simulink model "test_mdl"  (R2018a)
settings: Solver=VariableStepAuto  StartTime=0.0  StopTime=10.0  RelTol=1e-3
(part 4 of 8)

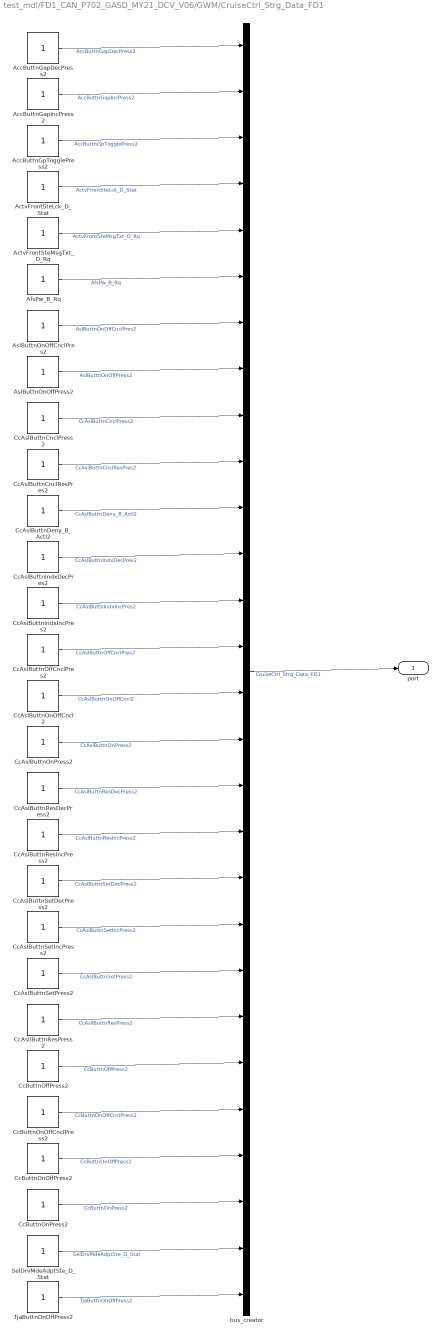
== system test_mdl/FD1_CAN_P702_GASD_MY21_DCV_V06/GWM/CruiseCtrl_Strg_Data_FD1 ==
  AccButtnGapDecPress2 : Constant
  AccButtnGapIncPress2 : Constant
  AccButtnGpTogglePress2 : Constant
  ActvFrontSteLck_D_Stat : Constant
  ActvFrontSteMsgTxt_D_Rq : Constant
  AfsPw_B_Rq : Constant
  AslButtnOnOffCnclPres2 : Constant
  AslButtnOnOffPress2 : Constant
  CcAslButtnCnclPress2 : Constant
  CcAslButtnCnclResPres2 : Constant
  CcAslButtnDeny_B_Actl2 : Constant
  CcAslButtnIndxDecPres2 : Constant
  CcAslButtnIndxIncPres2 : Constant
  CcAslButtnOffCnclPres2 : Constant
  CcAslButtnOnOffCncl2 : Constant
  CcAslButtnOnPress2 : Constant
  CcAslButtnResDecPress2 : Constant
  CcAslButtnResIncPress2 : Constant
  CcAslButtnSetDecPress2 : Constant
  CcAslButtnSetIncPress2 : Constant
  CcAslButtnSetPress2 : Constant
  CcAsllButtnResPress2 : Constant
  CcButtnOffPress2 : Constant
  CcButtnOnOffCnclPress2 : Constant
  CcButtnOnOffPress2 : Constant
  CcButtnOnPress2 : Constant
  SelDrvMdeAdptSte_D_Stat : Constant
  TjaButtnOnOffPress2 : Constant
  bus_creator : BusCreator  Inputs=28
  port : Outport
  wires:
  bus_creator/1 -> port/1  "CruiseCtrl_Strg_Data_FD1"
  AccButtnGapDecPress2/1 -> bus_creator/1  "AccButtnGapDecPress2"
  AccButtnGapIncPress2/1 -> bus_creator/2  "AccButtnGapIncPress2"
  AccButtnGpTogglePress2/1 -> bus_creator/3  "AccButtnGpTogglePress2"
  ActvFrontSteLck_D_Stat/1 -> bus_creator/4  "ActvFrontSteLck_D_Stat"
  ActvFrontSteMsgTxt_D_Rq/1 -> bus_creator/5  "ActvFrontSteMsgTxt_D_Rq"
  AfsPw_B_Rq/1 -> bus_creator/6  "AfsPw_B_Rq"
  AslButtnOnOffCnclPres2/1 -> bus_creator/7  "AslButtnOnOffCnclPres2"
  AslButtnOnOffPress2/1 -> bus_creator/8  "AslButtnOnOffPress2"
  CcAslButtnCnclPress2/1 -> bus_creator/9  "CcAslButtnCnclPress2"
  CcAslButtnCnclResPres2/1 -> bus_creator/10  "CcAslButtnCnclResPres2"
  CcAslButtnDeny_B_Actl2/1 -> bus_creator/11  "CcAslButtnDeny_B_Actl2"
  CcAslButtnIndxDecPres2/1 -> bus_creator/12  "CcAslButtnIndxDecPres2"
  CcAslButtnIndxIncPres2/1 -> bus_creator/13  "CcAslButtnIndxIncPres2"
  CcAslButtnOffCnclPres2/1 -> bus_creator/14  "CcAslButtnOffCnclPres2"
  CcAslButtnOnOffCncl2/1 -> bus_creator/15  "CcAslButtnOnOffCncl2"
  CcAslButtnOnPress2/1 -> bus_creator/16  "CcAslButtnOnPress2"
  CcAslButtnResDecPress2/1 -> bus_creator/17  "CcAslButtnResDecPress2"
  CcAslButtnResIncPress2/1 -> bus_creator/18  "CcAslButtnResIncPress2"
  CcAslButtnSetDecPress2/1 -> bus_creator/19  "CcAslButtnSetDecPress2"
  CcAslButtnSetIncPress2/1 -> bus_creator/20  "CcAslButtnSetIncPress2"
  CcAslButtnSetPress2/1 -> bus_creator/21  "CcAslButtnSetPress2"
  CcAsllButtnResPress2/1 -> bus_creator/22  "CcAsllButtnResPress2"
  CcButtnOffPress2/1 -> bus_creator/23  "CcButtnOffPress2"
  CcButtnOnOffCnclPress2/1 -> bus_creator/24  "CcButtnOnOffCnclPress2"
  CcButtnOnOffPress2/1 -> bus_creator/25  "CcButtnOnOffPress2"
  CcButtnOnPress2/1 -> bus_creator/26  "CcButtnOnPress2"
  SelDrvMdeAdptSte_D_Stat/1 -> bus_creator/27  "SelDrvMdeAdptSte_D_Stat"
  TjaButtnOnOffPress2/1 -> bus_creator/28  "TjaButtnOnOffPress2"

== system test_mdl/FD1_CAN_P702_GASD_MY21_DCV_V06/GWM/DCACA_Data1_FD1 ==
  CoolFanDcac_D_Rq : Constant
  DcacAcUDetct_B_Falt : Constant
  DcacBp1BrkrOpn_B_Falt : Constant
  DcacBp2BrkrOpn_B_Falt : Constant
  DcacClntFlw_D_Rq : Constant
  DcacErr_B_Stat : Constant
  DcacGfci_B_Falt : Constant
  DcacIpRcBrkrOpn_B_Falt : Constant
  DcacOverTe_B_Falt : Constant
  DcacOvrld_B_Falt : Constant
  DcacPlugPrsnt_B_Stat : Constant
  DcacRdy_D2_Stat : Constant
  DcacRdy_D_Stat : Constant
  bus_creator : BusCreator  Inputs=13
  port : Outport
  wires:
  bus_creator/1 -> port/1  "DCACA_Data1_FD1"
  CoolFanDcac_D_Rq/1 -> bus_creator/1  "CoolFanDcac_D_Rq"
  DcacAcUDetct_B_Falt/1 -> bus_creator/2  "DcacAcUDetct_B_Falt"
  DcacBp1BrkrOpn_B_Falt/1 -> bus_creator/3  "DcacBp1BrkrOpn_B_Falt"
  DcacBp2BrkrOpn_B_Falt/1 -> bus_creator/4  "DcacBp2BrkrOpn_B_Falt"
  DcacClntFlw_D_Rq/1 -> bus_creator/5  "DcacClntFlw_D_Rq"
  DcacErr_B_Stat/1 -> bus_creator/6  "DcacErr_B_Stat"
  DcacGfci_B_Falt/1 -> bus_creator/7  "DcacGfci_B_Falt"
  DcacIpRcBrkrOpn_B_Falt/1 -> bus_creator/8  "DcacIpRcBrkrOpn_B_Falt"
  DcacOverTe_B_Falt/1 -> bus_creator/9  "DcacOverTe_B_Falt"
  DcacOvrld_B_Falt/1 -> bus_creator/10  "DcacOvrld_B_Falt"
  DcacPlugPrsnt_B_Stat/1 -> bus_creator/11  "DcacPlugPrsnt_B_Stat"
  DcacRdy_D2_Stat/1 -> bus_creator/12  "DcacRdy_D2_Stat"
  DcacRdy_D_Stat/1 -> bus_creator/13  "DcacRdy_D_Stat"

== system test_mdl/FD1_CAN_P702_GASD_MY21_DCV_V06/GWM/DCACA_Data2_FD1 ==
  DcacIn_I_Actl : Constant
  DcacIn_U2_Actl : Constant
  DcacIn_U_Actl : Constant
  Dcac_Te_Actl : Constant
  bus_creator : BusCreator  Inputs=4
  port : Outport
  wires:
  bus_creator/1 -> port/1  "DCACA_Data2_FD1"
  DcacIn_I_Actl/1 -> bus_creator/1  "DcacIn_I_Actl"
  DcacIn_U2_Actl/1 -> bus_creator/2  "DcacIn_U2_Actl"
  DcacIn_U_Actl/1 -> bus_creator/3  "DcacIn_U_Actl"
  Dcac_Te_Actl/1 -> bus_creator/4  "Dcac_Te_Actl"

== system test_mdl/FD1_CAN_P702_GASD_MY21_DCV_V06/GWM/DCACA_Data3_FD1 ==
  DcacIn_Pw_Mx : Constant
  DcacOut1_Pw_Actl : Constant
  DcacOut2_Pw_Actl : Constant
  DcacOut_Pw_Mx : Constant
  bus_creator : BusCreator  Inputs=4
  port : Outport
  wires:
  bus_creator/1 -> port/1  "DCACA_Data3_FD1"
  DcacIn_Pw_Mx/1 -> bus_creator/1  "DcacIn_Pw_Mx"
  DcacOut1_Pw_Actl/1 -> bus_creator/2  "DcacOut1_Pw_Actl"
  DcacOut2_Pw_Actl/1 -> bus_creator/3  "DcacOut2_Pw_Actl"
  DcacOut_Pw_Mx/1 -> bus_creator/4  "DcacOut_Pw_Mx"

== system test_mdl/FD1_CAN_P702_GASD_MY21_DCV_V06/GWM/DTE_ECGtoHPCM ==
  DteCldBattULo_Eff_Actl : Constant
  DteCldClimt_Eff_Actl : Constant
  DteCldDcac_B_Stat : Constant
  DteCldDrv_Eff_Actl : Constant
  DteCldExtTe_B_Stat : Constant
  DteCldExt_Eff_Actl : Constant
  DteCldId_No_Actl : Constant
  DteCldPayload_B_Stat : Constant
  DteCldRoute_B_Stat : Constant
  DteCldTerrain_B_Stat : Constant
  DteCldTraffic_B_Stat : Constant
  DteCldTrip_L_Actl : Constant
  DteCldTrlrOff_B_Stat : Constant
  DteCldTrlrOn_B_Stat : Constant
  bus_creator : BusCreator  Inputs=14
  port : Outport
  wires:
  bus_creator/1 -> port/1  "DTE_ECGtoHPCM"
  DteCldBattULo_Eff_Actl/1 -> bus_creator/1  "DteCldBattULo_Eff_Actl"
  DteCldClimt_Eff_Actl/1 -> bus_creator/2  "DteCldClimt_Eff_Actl"
  DteCldDcac_B_Stat/1 -> bus_creator/3  "DteCldDcac_B_Stat"
  DteCldDrv_Eff_Actl/1 -> bus_creator/4  "DteCldDrv_Eff_Actl"
  DteCldExtTe_B_Stat/1 -> bus_creator/5  "DteCldExtTe_B_Stat"
  DteCldExt_Eff_Actl/1 -> bus_creator/6  "DteCldExt_Eff_Actl"
  DteCldId_No_Actl/1 -> bus_creator/7  "DteCldId_No_Actl"
  DteCldPayload_B_Stat/1 -> bus_creator/8  "DteCldPayload_B_Stat"
  DteCldRoute_B_Stat/1 -> bus_creator/9  "DteCldRoute_B_Stat"
  DteCldTerrain_B_Stat/1 -> bus_creator/10  "DteCldTerrain_B_Stat"
  DteCldTraffic_B_Stat/1 -> bus_creator/11  "DteCldTraffic_B_Stat"
  DteCldTrip_L_Actl/1 -> bus_creator/12  "DteCldTrip_L_Actl"
  DteCldTrlrOff_B_Stat/1 -> bus_creator/13  "DteCldTrlrOff_B_Stat"
  DteCldTrlrOn_B_Stat/1 -> bus_creator/14  "DteCldTrlrOn_B_Stat"

== system test_mdl/FD1_CAN_P702_GASD_MY21_DCV_V06/GWM/Driver_Dr_Stat_FD1 ==
  BLISLEDStatDriverSide : Constant
  ChildLckFdbckRd_B_Stat : Constant
  ChildLckPw_D_Rq : Constant
  ChildLckPw_N_Cnt : Constant
  Driver_Lock_Sw_Cnt : Constant
  Driver_Lock_Sw_Stat : Constant
  KeyCylSwDrvDr_D_Stat : Constant
  RollCodeDrvDrKeyCyl : Constant
  RvrseMirrorChime_B_Rq : Constant
  WndwDrvSide_D_Stat : Constant
  bus_creator : BusCreator  Inputs=10
  port : Outport
  wires:
  bus_creator/1 -> port/1  "Driver_Dr_Stat_FD1"
  BLISLEDStatDriverSide/1 -> bus_creator/1  "BLISLEDStatDriverSide"
  ChildLckFdbckRd_B_Stat/1 -> bus_creator/2  "ChildLckFdbckRd_B_Stat"
  ChildLckPw_D_Rq/1 -> bus_creator/3  "ChildLckPw_D_Rq"
  ChildLckPw_N_Cnt/1 -> bus_creator/4  "ChildLckPw_N_Cnt"
  Driver_Lock_Sw_Cnt/1 -> bus_creator/5  "Driver_Lock_Sw_Cnt"
  Driver_Lock_Sw_Stat/1 -> bus_creator/6  "Driver_Lock_Sw_Stat"
  KeyCylSwDrvDr_D_Stat/1 -> bus_creator/7  "KeyCylSwDrvDr_D_Stat"
  RollCodeDrvDrKeyCyl/1 -> bus_creator/8  "RollCodeDrvDrKeyCyl"
  RvrseMirrorChime_B_Rq/1 -> bus_creator/9  "RvrseMirrorChime_B_Rq"
  WndwDrvSide_D_Stat/1 -> bus_creator/10  "WndwDrvSide_D_Stat"

== system test_mdl/FD1_CAN_P702_GASD_MY21_DCV_V06/GWM/Dsp_Request_Signals11_FD1 ==
  ApaMdeStat_D_RqDrv : Constant
  ApaSwtch_D_RqMnu : Constant
  CamAutoTowbarZoom : Constant
  CamraOvrlDyn_D_Rq : Constant
  CamraOvrlStat_D_Rq : Constant
  CamraViewSplit_B_Rq : Constant
  CamraZoomMan_D_Rq : Constant
  DistanceBarSetting : Constant
  PrkAidSwtch_D_RqMnu : Constant
  bus_creator : BusCreator  Inputs=9
  port : Outport
  wires:
  bus_creator/1 -> port/1  "Dsp_Request_Signals11_FD1"
  ApaMdeStat_D_RqDrv/1 -> bus_creator/1  "ApaMdeStat_D_RqDrv"
  ApaSwtch_D_RqMnu/1 -> bus_creator/2  "ApaSwtch_D_RqMnu"
  CamAutoTowbarZoom/1 -> bus_creator/3  "CamAutoTowbarZoom"
  CamraOvrlDyn_D_Rq/1 -> bus_creator/4  "CamraOvrlDyn_D_Rq"
  CamraOvrlStat_D_Rq/1 -> bus_creator/5  "CamraOvrlStat_D_Rq"
  CamraViewSplit_B_Rq/1 -> bus_creator/6  "CamraViewSplit_B_Rq"
  CamraZoomMan_D_Rq/1 -> bus_creator/7  "CamraZoomMan_D_Rq"
  DistanceBarSetting/1 -> bus_creator/8  "DistanceBarSetting"
  PrkAidSwtch_D_RqMnu/1 -> bus_creator/9  "PrkAidSwtch_D_RqMnu"

== system test_mdl/FD1_CAN_P702_GASD_MY21_DCV_V06/GWM/ECG_Data2_FD1 ==
  DataMntrSustn_B_Rq : Constant
  DgtlCommPncReset_B_Req : Constant
  PwSustnRdata_B_RqTelem : Constant
  bus_creator : BusCreator  Inputs=3
  port : Outport
  wires:
  bus_creator/1 -> port/1  "ECG_Data2_FD1"
  DataMntrSustn_B_Rq/1 -> bus_creator/1  "DataMntrSustn_B_Rq"
  DgtlCommPncReset_B_Req/1 -> bus_creator/2  "DgtlCommPncReset_B_Req"
  PwSustnRdata_B_RqTelem/1 -> bus_creator/3  "PwSustnRdata_B_RqTelem"

== system test_mdl/FD1_CAN_P702_GASD_MY21_DCV_V06/GWM/ECG_Data3_FD1 ==
  BattULoChrg_D_RqOta : Constant
  CanMsg375_No_Cnt : Constant
  CanMsg375_No_Crc : Constant
  OtaActv_D_Stat : Constant
  VehOnRqstr_D_Stat : Constant
  VehOn_D_RqCld : Constant
  VehStrtInhbt_D_Dsply : Constant
  VehStrtInhbt_D_RqCld : Constant
  VehStrtInhbt_T_Dsply : Constant
  bus_creator : BusCreator  Inputs=9
  port : Outport
  wires:
  bus_creator/1 -> port/1  "ECG_Data3_FD1"
  BattULoChrg_D_RqOta/1 -> bus_creator/1  "BattULoChrg_D_RqOta"
  CanMsg375_No_Cnt/1 -> bus_creator/2  "CanMsg375_No_Cnt"
  CanMsg375_No_Crc/1 -> bus_creator/3  "CanMsg375_No_Crc"
  OtaActv_D_Stat/1 -> bus_creator/4  "OtaActv_D_Stat"
  VehOnRqstr_D_Stat/1 -> bus_creator/5  "VehOnRqstr_D_Stat"
  VehOn_D_RqCld/1 -> bus_creator/6  "VehOn_D_RqCld"
  VehStrtInhbt_D_Dsply/1 -> bus_creator/7  "VehStrtInhbt_D_Dsply"
  VehStrtInhbt_D_RqCld/1 -> bus_creator/8  "VehStrtInhbt_D_RqCld"
  VehStrtInhbt_T_Dsply/1 -> bus_creator/9  "VehStrtInhbt_T_Dsply"

== system test_mdl/FD1_CAN_P702_GASD_MY21_DCV_V06/GWM/ECG_Data4_FD1 ==
  PtWakeupActv1_B_Rq : Constant
  bus_creator : BusCreator  Inputs=1
  port : Outport
  wires:
  bus_creator/1 -> port/1  "ECG_Data4_FD1"
  PtWakeupActv1_B_Rq/1 -> bus_creator/1  "PtWakeupActv1_B_Rq"

== system test_mdl/FD1_CAN_P702_GASD_MY21_DCV_V06/GWM/ECG_Data_FD1 ==
  ChrgrPncEnbl_D_Rq : Constant
  ChrgrPncSustn_B_Rq : Constant
  ExtLghtDsply_B_StatArb : Constant
  ExtLghtFront_D_RqOta : Constant
  ExtLghtLeft_D_RqOta : Constant
  ExtLghtRear_D_RqOta : Constant
  ExtLghtRight_D_RqOta : Constant
  NtfyDrvSocLvl1_Pc_Rq : Constant
  NtfyDrvTrgtDist_L_Rq : Constant
  OBCCSerial_D_Rq : Constant
  PtRmtRprt_D_Stat : Constant
  TlghtTest_D_RqArb : Constant
  bus_creator : BusCreator  Inputs=12
  port : Outport
  wires:
  bus_creator/1 -> port/1  "ECG_Data_FD1"
  ChrgrPncEnbl_D_Rq/1 -> bus_creator/1  "ChrgrPncEnbl_D_Rq"
  ChrgrPncSustn_B_Rq/1 -> bus_creator/2  "ChrgrPncSustn_B_Rq"
  ExtLghtDsply_B_StatArb/1 -> bus_creator/3  "ExtLghtDsply_B_StatArb"
  ExtLghtFront_D_RqOta/1 -> bus_creator/4  "ExtLghtFront_D_RqOta"
  ExtLghtLeft_D_RqOta/1 -> bus_creator/5  "ExtLghtLeft_D_RqOta"
  ExtLghtRear_D_RqOta/1 -> bus_creator/6  "ExtLghtRear_D_RqOta"
  ExtLghtRight_D_RqOta/1 -> bus_creator/7  "ExtLghtRight_D_RqOta"
  NtfyDrvSocLvl1_Pc_Rq/1 -> bus_creator/8  "NtfyDrvSocLvl1_Pc_Rq"
  NtfyDrvTrgtDist_L_Rq/1 -> bus_creator/9  "NtfyDrvTrgtDist_L_Rq"
  OBCCSerial_D_Rq/1 -> bus_creator/10  "OBCCSerial_D_Rq"
  PtRmtRprt_D_Stat/1 -> bus_creator/11  "PtRmtRprt_D_Stat"
  TlghtTest_D_RqArb/1 -> bus_creator/12  "TlghtTest_D_RqArb"

== system test_mdl/FD1_CAN_P702_GASD_MY21_DCV_V06/GWM/ElecHorizon_Data1_FD1 ==
  EhData1_No_Actl : Constant
  bus_creator : BusCreator  Inputs=1
  port : Outport
  wires:
  bus_creator/1 -> port/1  "ElecHorizon_Data1_FD1"
  EhData1_No_Actl/1 -> bus_creator/1  "EhData1_No_Actl"

== system test_mdl/FD1_CAN_P702_GASD_MY21_DCV_V06/GWM/ElecHorizon_Data2_FD1 ==
  EhData2_No_Actl : Constant
  bus_creator : BusCreator  Inputs=1
  port : Outport
  wires:
  bus_creator/1 -> port/1  "ElecHorizon_Data2_FD1"
  EhData2_No_Actl/1 -> bus_creator/1  "EhData2_No_Actl"

== system test_mdl/FD1_CAN_P702_GASD_MY21_DCV_V06/GWM/FourByFourSwitchData_FD1 ==
  AwdMde_D_RqDrv : Constant
  DrvSlipCtlMde_B_Rq3 : Constant
  HdcSwtchPos_B_Actl : Constant
  HybMdeSwtch_B_Rq : Constant
  RearDiffLck_D_RqDrv : Constant
  TrailCtlSwtch_B_Stat3 : Constant
  bus_creator : BusCreator  Inputs=6
  port : Outport
  wires:
  bus_creator/1 -> port/1  "FourByFourSwitchData_FD1"
  AwdMde_D_RqDrv/1 -> bus_creator/1  "AwdMde_D_RqDrv"
  DrvSlipCtlMde_B_Rq3/1 -> bus_creator/2  "DrvSlipCtlMde_B_Rq3"
  HdcSwtchPos_B_Actl/1 -> bus_creator/3  "HdcSwtchPos_B_Actl"
  HybMdeSwtch_B_Rq/1 -> bus_creator/4  "HybMdeSwtch_B_Rq"
  RearDiffLck_D_RqDrv/1 -> bus_creator/5  "RearDiffLck_D_RqDrv"
  TrailCtlSwtch_B_Stat3/1 -> bus_creator/6  "TrailCtlSwtch_B_Stat3"

== system test_mdl/FD1_CAN_P702_GASD_MY21_DCV_V06/GWM/GGCC_Config_Mgmt_ID_1_FD1 ==
  VehicleGGCCData : Constant
  bus_creator : BusCreator  Inputs=1
  port : Outport
  wires:
  bus_creator/1 -> port/1  "GGCC_Config_Mgmt_ID_1_FD1"
  VehicleGGCCData/1 -> bus_creator/1  "VehicleGGCCData"

== system test_mdl/FD1_CAN_P702_GASD_MY21_DCV_V06/GWM/GWM_AutoSar_NetMgmt_FD1 ==
  GWM_AutoSarNMControl : Constant
  GWM_AutoSarNMNodeId : Constant
  GWM_AutoSarNMReserved{1..4} (4 alike) : Constant
  GWM_GWNMProxy : Constant
  GWM_GWOnBoardTester : Constant
  bus_creator : BusCreator  Inputs=8
  port : Outport
  wires:
  bus_creator/1 -> port/1  "GWM_AutoSar_NetMgmt_FD1"
  GWM_AutoSarNMControl/1 -> bus_creator/1  "GWM_AutoSarNMControl"
  GWM_AutoSarNMNodeId/1 -> bus_creator/2  "GWM_AutoSarNMNodeId"
  GWM_AutoSarNMReserved1/1 -> bus_creator/3  "GWM_AutoSarNMReserved1"
  GWM_AutoSarNMReserved2/1 -> bus_creator/4  "GWM_AutoSarNMReserved2"
  GWM_AutoSarNMReserved3/1 -> bus_creator/5  "GWM_AutoSarNMReserved3"
  GWM_AutoSarNMReserved4/1 -> bus_creator/6  "GWM_AutoSarNMReserved4"
  GWM_GWNMProxy/1 -> bus_creator/7  "GWM_GWNMProxy"
  GWM_GWOnBoardTester/1 -> bus_creator/8  "GWM_GWOnBoardTester"

== system test_mdl/FD1_CAN_P702_GASD_MY21_DCV_V06/GWM/Gear_Shift_by_Wire_2_FD1 ==
  GearButtnStuck_B_Actl : Constant
  GsmSrvcRqd_B_Rq : Constant
  TrnGearPwmFalt_B_Actl : Constant
  bus_creator : BusCreator  Inputs=3
  port : Outport
  wires:
  bus_creator/1 -> port/1  "Gear_Shift_by_Wire_2_FD1"
  GearButtnStuck_B_Actl/1 -> bus_creator/1  "GearButtnStuck_B_Actl"
  GsmSrvcRqd_B_Rq/1 -> bus_creator/2  "GsmSrvcRqd_B_Rq"
  TrnGearPwmFalt_B_Actl/1 -> bus_creator/3  "TrnGearPwmFalt_B_Actl"

== system test_mdl/FD1_CAN_P702_GASD_MY21_DCV_V06/GWM/Gear_Shift_by_Wire_FD1 ==
  BrkSwtchPos_B_ActlGsm : Constant
  DrQltyDrv_D_StatGsm : Constant
  GsmGearMsgTxt_D_Rq : Constant
  PrkBrkActv_D_RqGsmGear : Constant
  TrnBtsiOvrrd_B_Stat : Constant
  TrnGearButtn_B_ActlD0 : Constant
  TrnGearButtn_B_ActlD1 : Constant
  TrnGearButtn_B_ActlD2 : Constant
  TrnGearButtn_B_ActlM0 : Constant
  TrnGearButtn_B_ActlM1 : Constant
  TrnGearButtn_B_ActlM2 : Constant
  TrnGearButtn_B_ActlN0 : Constant
  TrnGearButtn_B_ActlN1 : Constant
  TrnGearButtn_B_ActlN2 : Constant
  TrnGearButtn_B_ActlP0 : Constant
  TrnGearButtn_B_ActlP1 : Constant
  TrnGearButtn_B_ActlP2 : Constant
  TrnGearButtn_B_ActlR0 : Constant
  TrnGearButtn_B_ActlR1 : Constant
  TrnGearButtn_B_ActlR2 : Constant
  TrnGearButtn_U_Actl : Constant
  TrnGearRqCnt_B_Actl : Constant
  TrnGear_D_RqDrv : Constant
  TrnGear_No_Cnt : Constant
  TrnGear_No_Cs : Constant
  TrnGsmNtmState_D_Actl : Constant
  TrnRng_D_RqGsm : Constant
  TrnValidGearRq_D_Stat : Constant
  bus_creator : BusCreator  Inputs=28
  port : Outport
  wires:
  bus_creator/1 -> port/1  "Gear_Shift_by_Wire_FD1"
  BrkSwtchPos_B_ActlGsm/1 -> bus_creator/1  "BrkSwtchPos_B_ActlGsm"
  DrQltyDrv_D_StatGsm/1 -> bus_creator/2  "DrQltyDrv_D_StatGsm"
  GsmGearMsgTxt_D_Rq/1 -> bus_creator/3  "GsmGearMsgTxt_D_Rq"
  PrkBrkActv_D_RqGsmGear/1 -> bus_creator/4  "PrkBrkActv_D_RqGsmGear"
  TrnBtsiOvrrd_B_Stat/1 -> bus_creator/5  "TrnBtsiOvrrd_B_Stat"
  TrnGearButtn_B_ActlD0/1 -> bus_creator/6  "TrnGearButtn_B_ActlD0"
  TrnGearButtn_B_ActlD1/1 -> bus_creator/7  "TrnGearButtn_B_ActlD1"
  TrnGearButtn_B_ActlD2/1 -> bus_creator/8  "TrnGearButtn_B_ActlD2"
  TrnGearButtn_B_ActlM0/1 -> bus_creator/9  "TrnGearButtn_B_ActlM0"
  TrnGearButtn_B_ActlM1/1 -> bus_creator/10  "TrnGearButtn_B_ActlM1"
  TrnGearButtn_B_ActlM2/1 -> bus_creator/11  "TrnGearButtn_B_ActlM2"
  TrnGearButtn_B_ActlN0/1 -> bus_creator/12  "TrnGearButtn_B_ActlN0"
  TrnGearButtn_B_ActlN1/1 -> bus_creator/13  "TrnGearButtn_B_ActlN1"
  TrnGearButtn_B_ActlN2/1 -> bus_creator/14  "TrnGearButtn_B_ActlN2"
  TrnGearButtn_B_ActlP0/1 -> bus_creator/15  "TrnGearButtn_B_ActlP0"
  TrnGearButtn_B_ActlP1/1 -> bus_creator/16  "TrnGearButtn_B_ActlP1"
  TrnGearButtn_B_ActlP2/1 -> bus_creator/17  "TrnGearButtn_B_ActlP2"
  TrnGearButtn_B_ActlR0/1 -> bus_creator/18  "TrnGearButtn_B_ActlR0"
  TrnGearButtn_B_ActlR1/1 -> bus_creator/19  "TrnGearButtn_B_ActlR1"
  TrnGearButtn_B_ActlR2/1 -> bus_creator/20  "TrnGearButtn_B_ActlR2"
  TrnGearButtn_U_Actl/1 -> bus_creator/21  "TrnGearButtn_U_Actl"
  TrnGearRqCnt_B_Actl/1 -> bus_creator/22  "TrnGearRqCnt_B_Actl"
  TrnGear_D_RqDrv/1 -> bus_creator/23  "TrnGear_D_RqDrv"
  TrnGear_No_Cnt/1 -> bus_creator/24  "TrnGear_No_Cnt"
  TrnGear_No_Cs/1 -> bus_creator/25  "TrnGear_No_Cs"
  TrnGsmNtmState_D_Actl/1 -> bus_creator/26  "TrnGsmNtmState_D_Actl"
  TrnRng_D_RqGsm/1 -> bus_creator/27  "TrnRng_D_RqGsm"
  TrnValidGearRq_D_Stat/1 -> bus_creator/28  "TrnValidGearRq_D_Stat"

== system test_mdl/FD1_CAN_P702_GASD_MY21_DCV_V06/GWM/GlobalClock_Data_FD1 ==
  GlblClkDay_No_Actl : Constant
  GlblClkHr_No_Actl : Constant
  GlblClkMnte_No_Actl : Constant
  GlblClkScnd_No_Actl : Constant
  GlblClkYr_No_Actl : Constant
  bus_creator : BusCreator  Inputs=5
  port : Outport
  wires:
  bus_creator/1 -> port/1  "GlobalClock_Data_FD1"
  GlblClkDay_No_Actl/1 -> bus_creator/1  "GlblClkDay_No_Actl"
  GlblClkHr_No_Actl/1 -> bus_creator/2  "GlblClkHr_No_Actl"
  GlblClkMnte_No_Actl/1 -> bus_creator/3  "GlblClkMnte_No_Actl"
  GlblClkScnd_No_Actl/1 -> bus_creator/4  "GlblClkScnd_No_Actl"
  GlblClkYr_No_Actl/1 -> bus_creator/5  "GlblClkYr_No_Actl"

== system test_mdl/FD1_CAN_P702_GASD_MY21_DCV_V06/GWM/Global_PATS_Cntrl_Info_FD1 ==
  bus_creator : BusCreator  Inputs=2
  immoControlCmd_T1 : Constant
  immoControlData_T1 : Constant
  port : Outport
  wires:
  bus_creator/1 -> port/1  "Global_PATS_Cntrl_Info_FD1"
  immoControlCmd_T1/1 -> bus_creator/1  "immoControlCmd_T1"
  immoControlData_T1/1 -> bus_creator/2  "immoControlData_T1"

== system test_mdl/FD1_CAN_P702_GASD_MY21_DCV_V06/GWM/Global_PATS_Ctrl_Info2_FD1 ==
  bus_creator : BusCreator  Inputs=2
  immoControlCmd_T2 : Constant
  immoControlData_T2 : Constant
  port : Outport
  wires:
  bus_creator/1 -> port/1  "Global_PATS_Ctrl_Info2_FD1"
  immoControlCmd_T2/1 -> bus_creator/1  "immoControlCmd_T2"
  immoControlData_T2/1 -> bus_creator/2  "immoControlData_T2"

== system test_mdl/FD1_CAN_P702_GASD_MY21_DCV_V06/GWM/HeadUpDisplayReq_FD1 ==
  SelDrvMdeCnfm_D_Stat : Constant
  bus_creator : BusCreator  Inputs=1
  port : Outport
  wires:
  bus_creator/1 -> port/1  "HeadUpDisplayReq_FD1"
  SelDrvMdeCnfm_D_Stat/1 -> bus_creator/1  "SelDrvMdeCnfm_D_Stat"

== system test_mdl/FD1_CAN_P702_GASD_MY21_DCV_V06/GWM/IPC_Infotainment_FD1 ==
  BeltminderAudioMute : Constant
  Chime_Source : Constant
  HdcOn_B_Rq : Constant
  IPC_Attn_Info_Audio : Constant
  IPC_MyKeyVolLimit_St : Constant
  IPC_New_Attn_Event : Constant
  Power_Up_Chime_Modules : Constant
  Veh_V2_Dsply : Constant
  bus_creator : BusCreator  Inputs=8
  port : Outport
  wires:
  bus_creator/1 -> port/1  "IPC_Infotainment_FD1"
  BeltminderAudioMute/1 -> bus_creator/1  "BeltminderAudioMute"
  Chime_Source/1 -> bus_creator/2  "Chime_Source"
  HdcOn_B_Rq/1 -> bus_creator/3  "HdcOn_B_Rq"
  IPC_Attn_Info_Audio/1 -> bus_creator/4  "IPC_Attn_Info_Audio"
  IPC_MyKeyVolLimit_St/1 -> bus_creator/5  "IPC_MyKeyVolLimit_St"
  IPC_New_Attn_Event/1 -> bus_creator/6  "IPC_New_Attn_Event"
  Power_Up_Chime_Modules/1 -> bus_creator/7  "Power_Up_Chime_Modules"
  Veh_V2_Dsply/1 -> bus_creator/8  "Veh_V2_Dsply"

== system test_mdl/FD1_CAN_P702_GASD_MY21_DCV_V06/GWM/IPC_Send_Signals_2_FD1 ==
  ElLongTerm_L_Dsply : Constant
  ElTrip_L_Dsply : Constant
  FuelRange_L_Dsply : Constant
  bus_creator : BusCreator  Inputs=3
  port : Outport
  wires:
  bus_creator/1 -> port/1  "IPC_Send_Signals_2_FD1"
  ElLongTerm_L_Dsply/1 -> bus_creator/1  "ElLongTerm_L_Dsply"
  ElTrip_L_Dsply/1 -> bus_creator/2  "ElTrip_L_Dsply"
  FuelRange_L_Dsply/1 -> bus_creator/3  "FuelRange_L_Dsply"

== system test_mdl/FD1_CAN_P702_GASD_MY21_DCV_V06/GWM/LocationServices_3_FD1 ==
  LocationServices_3 : Constant
  bus_creator : BusCreator  Inputs=1
  port : Outport
  wires:
  bus_creator/1 -> port/1  "LocationServices_3_FD1"
  LocationServices_3/1 -> bus_creator/1  "LocationServices_3"

== system test_mdl/FD1_CAN_P702_GASD_MY21_DCV_V06/GWM/LocationServices_Data1_FD1 ==
  LocationServices_1 : Constant
  bus_creator : BusCreator  Inputs=1
  port : Outport
  wires:
  bus_creator/1 -> port/1  "LocationServices_Data1_FD1"
  LocationServices_1/1 -> bus_creator/1  "LocationServices_1"

== system test_mdl/FD1_CAN_P702_GASD_MY21_DCV_V06/GWM/Locking_Systems_2_FD1 ==
  ChildLckMde_B_Stat : Constant
  ChildLck_D_Dsply : Constant
  DrTgateExtSwMde_B_Stat : Constant
  DrTgateOpen_B_Rq : Constant
  FobComm_D_Stat : Constant
  Keyfob_Pad_Msg_Count : Constant
  L_Pwr_Sliding_Dr_Rqst : Constant
  LockInhibit : Constant
  Lockmsgtxt_D_Rq : Constant
  Power_Decklid_Rqst : Constant
  Power_Liftgate_Rqst : Constant
  R_Pwr_Sliding_Dr_Rqst : Constant
  Remote_Device_Feedback : Constant
  RollCodeUnlock : Constant
  VehLckInd_D_Rq : Constant
  Veh_Lock_EvNum : Constant
  Veh_Lock_Requestor : Constant
  Veh_Lock_Status : Constant
  Veh_Lock_Sub_Id : Constant
  WindowLockout_B_Stat : Constant
  bus_creator : BusCreator  Inputs=20
  port : Outport
  wires:
  bus_creator/1 -> port/1  "Locking_Systems_2_FD1"
  ChildLckMde_B_Stat/1 -> bus_creator/1  "ChildLckMde_B_Stat"
  ChildLck_D_Dsply/1 -> bus_creator/2  "ChildLck_D_Dsply"
  DrTgateExtSwMde_B_Stat/1 -> bus_creator/3  "DrTgateExtSwMde_B_Stat"
  DrTgateOpen_B_Rq/1 -> bus_creator/4  "DrTgateOpen_B_Rq"
  FobComm_D_Stat/1 -> bus_creator/5  "FobComm_D_Stat"
  Keyfob_Pad_Msg_Count/1 -> bus_creator/6  "Keyfob_Pad_Msg_Count"
  L_Pwr_Sliding_Dr_Rqst/1 -> bus_creator/7  "L_Pwr_Sliding_Dr_Rqst"
  LockInhibit/1 -> bus_creator/8  "LockInhibit"
  Lockmsgtxt_D_Rq/1 -> bus_creator/9  "Lockmsgtxt_D_Rq"
  Power_Decklid_Rqst/1 -> bus_creator/10  "Power_Decklid_Rqst"
  Power_Liftgate_Rqst/1 -> bus_creator/11  "Power_Liftgate_Rqst"
  R_Pwr_Sliding_Dr_Rqst/1 -> bus_creator/12  "R_Pwr_Sliding_Dr_Rqst"
  Remote_Device_Feedback/1 -> bus_creator/13  "Remote_Device_Feedback"
  RollCodeUnlock/1 -> bus_creator/14  "RollCodeUnlock"
  VehLckInd_D_Rq/1 -> bus_creator/15  "VehLckInd_D_Rq"
  Veh_Lock_EvNum/1 -> bus_creator/16  "Veh_Lock_EvNum"
  Veh_Lock_Requestor/1 -> bus_creator/17  "Veh_Lock_Requestor"
  Veh_Lock_Status/1 -> bus_creator/18  "Veh_Lock_Status"
  Veh_Lock_Sub_Id/1 -> bus_creator/19  "Veh_Lock_Sub_Id"
  WindowLockout_B_Stat/1 -> bus_creator/20  "WindowLockout_B_Stat"

== system test_mdl/FD1_CAN_P702_GASD_MY21_DCV_V06/GWM/MasterReset_HS3_ECGDat_FD1 ==
  DrvBhavWarn_B_Rq : Constant
  FactoryReset_St : Constant
  KeyOffPwMde_D_Stat : Constant
  ModemReset_D_Stat : Constant
  OfbChrgSetSync_D_Rq : Constant
  bus_creator : BusCreator  Inputs=5
  port : Outport
  wires:
  bus_creator/1 -> port/1  "MasterReset_HS3_ECGDat_FD1"
  DrvBhavWarn_B_Rq/1 -> bus_creator/1  "DrvBhavWarn_B_Rq"
  FactoryReset_St/1 -> bus_creator/2  "FactoryReset_St"
  KeyOffPwMde_D_Stat/1 -> bus_creator/3  "KeyOffPwMde_D_Stat"
  ModemReset_D_Stat/1 -> bus_creator/4  "ModemReset_D_Stat"
  OfbChrgSetSync_D_Rq/1 -> bus_creator/5  "OfbChrgSetSync_D_Rq"

== system test_mdl/FD1_CAN_P702_GASD_MY21_DCV_V06/GWM/Mc_Send_Signals_2_FD1 ==
  AwdRnge_D_ActlIpc : Constant
  BalrMde_D_Rq : Constant
  BalrSwtch_D_Stat : Constant
  BttOn_B_Rq : Constant
  Btt_L_Actl : Constant
  DrvInputRequired_B_Rq : Constant
  EdmSailMde_B_RqDrv : Constant
  EngExhMdeQuiet_D2_Rq : Constant
  EsaOn_B_Rq : Constant
  Mc_VehLangUsrSel_St : Constant
  Mc_VehTimeFrmtUsrSel_St : Constant
  Mc_VehUnitTempUsrSel_St : Constant
  Mc_VehUntTrpCoUsrSel_St : Constant
  Running_Board_Cmd : Constant
  SelDrvMdeDsply_B_Avail : Constant
  SelDrvMdeTxtReset_B_Rq : Constant
  WaitToStartLamp_D_Falt : Constant
  bus_creator : BusCreator  Inputs=17
  port : Outport
  wires:
  bus_creator/1 -> port/1  "Mc_Send_Signals_2_FD1"
  AwdRnge_D_ActlIpc/1 -> bus_creator/1  "AwdRnge_D_ActlIpc"
  BalrMde_D_Rq/1 -> bus_creator/2  "BalrMde_D_Rq"
  BalrSwtch_D_Stat/1 -> bus_creator/3  "BalrSwtch_D_Stat"
  BttOn_B_Rq/1 -> bus_creator/4  "BttOn_B_Rq"
  Btt_L_Actl/1 -> bus_creator/5  "Btt_L_Actl"
  DrvInputRequired_B_Rq/1 -> bus_creator/6  "DrvInputRequired_B_Rq"
  EdmSailMde_B_RqDrv/1 -> bus_creator/7  "EdmSailMde_B_RqDrv"
  EngExhMdeQuiet_D2_Rq/1 -> bus_creator/8  "EngExhMdeQuiet_D2_Rq"
  EsaOn_B_Rq/1 -> bus_creator/9  "EsaOn_B_Rq"
  Mc_VehLangUsrSel_St/1 -> bus_creator/10  "Mc_VehLangUsrSel_St"
  Mc_VehTimeFrmtUsrSel_St/1 -> bus_creator/11  "Mc_VehTimeFrmtUsrSel_St"
  Mc_VehUnitTempUsrSel_St/1 -> bus_creator/12  "Mc_VehUnitTempUsrSel_St"
  Mc_VehUntTrpCoUsrSel_St/1 -> bus_creator/13  "Mc_VehUntTrpCoUsrSel_St"
  Running_Board_Cmd/1 -> bus_creator/14  "Running_Board_Cmd"
  SelDrvMdeDsply_B_Avail/1 -> bus_creator/15  "SelDrvMdeDsply_B_Avail"
  SelDrvMdeTxtReset_B_Rq/1 -> bus_creator/16  "SelDrvMdeTxtReset_B_Rq"
  WaitToStartLamp_D_Falt/1 -> bus_creator/17  "WaitToStartLamp_D_Falt"

== system test_mdl/FD1_CAN_P702_GASD_MY21_DCV_V06/GWM/OTAFuncGWM_ECG_FD1 ==
  OTAFuncGWM_ECG : Constant
  bus_creator : BusCreator  Inputs=1
  port : Outport
  wires:
  bus_creator/1 -> port/1  "OTAFuncGWM_ECG_FD1"
  OTAFuncGWM_ECG/1 -> bus_creator/1  "OTAFuncGWM_ECG"

== system test_mdl/FD1_CAN_P702_GASD_MY21_DCV_V06/GWM/OTAPhysGWM_ECGtoABS ==
  OTAPhysGWM_ECGtoABS : Constant
  bus_creator : BusCreator  Inputs=1
  port : Outport
  wires:
  bus_creator/1 -> port/1  "OTAPhysGWM_ECGtoABS"
  OTAPhysGWM_ECGtoABS/1 -> bus_creator/1  "OTAPhysGWM_ECGtoABS"

== system test_mdl/FD1_CAN_P702_GASD_MY21_DCV_V06/GWM/OTAPhysGWM_ECGtoCCM ==
  OTAPhysGWM_ECGtoCCM : Constant
  bus_creator : BusCreator  Inputs=1
  port : Outport
  wires:
  bus_creator/1 -> port/1  "OTAPhysGWM_ECGtoCCM"
  OTAPhysGWM_ECGtoCCM/1 -> bus_creator/1  "OTAPhysGWM_ECGtoCCM"

== system test_mdl/FD1_CAN_P702_GASD_MY21_DCV_V06/GWM/OTAPhysGWM_ECGtoIPMA ==
  OTAPhysGWM_ECGtoIPMA : Constant
  bus_creator : BusCreator  Inputs=1
  port : Outport
  wires:
  bus_creator/1 -> port/1  "OTAPhysGWM_ECGtoIPMA"
  OTAPhysGWM_ECGtoIPMA/1 -> bus_creator/1  "OTAPhysGWM_ECGtoIPMA"

== system test_mdl/FD1_CAN_P702_GASD_MY21_DCV_V06/GWM/OTAPhysGWM_ECGtoPCM ==
  OTAPhysGWM_ECGtoPCM : Constant
  bus_creator : BusCreator  Inputs=1
  port : Outport
  wires:
  bus_creator/1 -> port/1  "OTAPhysGWM_ECGtoPCM"
  OTAPhysGWM_ECGtoPCM/1 -> bus_creator/1  "OTAPhysGWM_ECGtoPCM"

== system test_mdl/FD1_CAN_P702_GASD_MY21_DCV_V06/GWM/OTAPhysGWM_ECGtoSOBDMC_FD1 ==
  OTAPhysGWM_ECGtoHPCM : Constant
  bus_creator : BusCreator  Inputs=1
  port : Outport
  wires:
  bus_creator/1 -> port/1  "OTAPhysGWM_ECGtoSOBDMC_FD1"
  OTAPhysGWM_ECGtoHPCM/1 -> bus_creator/1  "OTAPhysGWM_ECGtoHPCM"

== system test_mdl/FD1_CAN_P702_GASD_MY21_DCV_V06/GWM/OTAPhysGWM_ECGtoSODCMC ==
  OTAPhysGWM_ECGtoSODCMC : Constant
  bus_creator : BusCreator  Inputs=1
  port : Outport
  wires:
  bus_creator/1 -> port/1  "OTAPhysGWM_ECGtoSODCMC"
  OTAPhysGWM_ECGtoSODCMC/1 -> bus_creator/1  "OTAPhysGWM_ECGtoSODCMC"

== system test_mdl/FD1_CAN_P702_GASD_MY21_DCV_V06/GWM/OTAPhysGWM_ECGtoSODCMD ==
  OTAPhysGWM_ECGtoSODCMD : Constant
  bus_creator : BusCreator  Inputs=1
  port : Outport
  wires:
  bus_creator/1 -> port/1  "OTAPhysGWM_ECGtoSODCMD"
  OTAPhysGWM_ECGtoSODCMD/1 -> bus_creator/1  "OTAPhysGWM_ECGtoSODCMD"

== system test_mdl/FD1_CAN_P702_GASD_MY21_DCV_V06/GWM/OTAPhysGWM_ECGtoSODL ==
  OTAPhysGWM_ECGtoSODL : Constant
  bus_creator : BusCreator  Inputs=1
  port : Outport
  wires:
  bus_creator/1 -> port/1  "OTAPhysGWM_ECGtoSODL"
  OTAPhysGWM_ECGtoSODL/1 -> bus_creator/1  "OTAPhysGWM_ECGtoSODL"

== system test_mdl/FD1_CAN_P702_GASD_MY21_DCV_V06/GWM/OTAPhysGWM_ECGtoSODR ==
  OTAPhysGWM_ECGtoSODR : Constant
  bus_creator : BusCreator  Inputs=1
  port : Outport
  wires:
  bus_creator/1 -> port/1  "OTAPhysGWM_ECGtoSODR"
  OTAPhysGWM_ECGtoSODR/1 -> bus_creator/1  "OTAPhysGWM_ECGtoSODR"

== system test_mdl/FD1_CAN_P702_GASD_MY21_DCV_V06/GWM/OffBrdChrg_Signals ==
  OfbChrgLocIdTrgt_No_Rq : Constant
  OfbChrgLocIdUns_B_Rq : Constant
  OfbChrgPrflWkdy_No_Rq : Constant
  OfbChrgPrflWknd_No_Rq : Constant
  OfbChrgSetDelete_B_Rq : Constant
  OfbChrgSetNow_D_Rq : Constant
  OfbChrgToPcWkdy_D_Actl : Constant
  OfbChrgToPcWknd_D_Actl : Constant
  bus_creator : BusCreator  Inputs=8
  port : Outport
  wires:
  bus_creator/1 -> port/1  "OffBrdChrg_Signals"
  OfbChrgLocIdTrgt_No_Rq/1 -> bus_creator/1  "OfbChrgLocIdTrgt_No_Rq"
  OfbChrgLocIdUns_B_Rq/1 -> bus_creator/2  "OfbChrgLocIdUns_B_Rq"
  OfbChrgPrflWkdy_No_Rq/1 -> bus_creator/3  "OfbChrgPrflWkdy_No_Rq"
  OfbChrgPrflWknd_No_Rq/1 -> bus_creator/4  "OfbChrgPrflWknd_No_Rq"
  OfbChrgSetDelete_B_Rq/1 -> bus_creator/5  "OfbChrgSetDelete_B_Rq"
  OfbChrgSetNow_D_Rq/1 -> bus_creator/6  "OfbChrgSetNow_D_Rq"
  OfbChrgToPcWkdy_D_Actl/1 -> bus_creator/7  "OfbChrgToPcWkdy_D_Actl"
  OfbChrgToPcWknd_D_Actl/1 -> bus_creator/8  "OfbChrgToPcWknd_D_Actl"

== system test_mdl/FD1_CAN_P702_GASD_MY21_DCV_V06/GWM/OffBrdChrg_Signals2 ==
  OfbChrgClearAll_B_Rq : Constant
  OfbChrgGoTDelete_B_Rq : Constant
  OfbChrgGoTElement_D_Rq : Constant
  OfbChrgGoTExtHtr_D_Rq : Constant
  OfbChrgGoTHr_T_Rq : Constant
  OfbChrgGoTMnte_D_Rq : Constant
  OfbChrgGoTOn_D_Rq : Constant
  OfbChrgGoTPrcond_D_Rq : Constant
  OfbChrgGoTTouch_D_Rq : Constant
  OfbChrgGoTUpdate_B_Rq : Constant
  OfbChrgPrflUpdate_B_Rq : Constant
  bus_creator : BusCreator  Inputs=11
  port : Outport
  wires:
  bus_creator/1 -> port/1  "OffBrdChrg_Signals2"
  OfbChrgClearAll_B_Rq/1 -> bus_creator/1  "OfbChrgClearAll_B_Rq"
  OfbChrgGoTDelete_B_Rq/1 -> bus_creator/2  "OfbChrgGoTDelete_B_Rq"
  OfbChrgGoTElement_D_Rq/1 -> bus_creator/3  "OfbChrgGoTElement_D_Rq"
  OfbChrgGoTExtHtr_D_Rq/1 -> bus_creator/4  "OfbChrgGoTExtHtr_D_Rq"
  OfbChrgGoTHr_T_Rq/1 -> bus_creator/5  "OfbChrgGoTHr_T_Rq"
  OfbChrgGoTMnte_D_Rq/1 -> bus_creator/6  "OfbChrgGoTMnte_D_Rq"
  OfbChrgGoTOn_D_Rq/1 -> bus_creator/7  "OfbChrgGoTOn_D_Rq"
  OfbChrgGoTPrcond_D_Rq/1 -> bus_creator/8  "OfbChrgGoTPrcond_D_Rq"
  OfbChrgGoTTouch_D_Rq/1 -> bus_creator/9  "OfbChrgGoTTouch_D_Rq"
  OfbChrgGoTUpdate_B_Rq/1 -> bus_creator/10  "OfbChrgGoTUpdate_B_Rq"
  OfbChrgPrflUpdate_B_Rq/1 -> bus_creator/11  "OfbChrgPrflUpdate_B_Rq"

== system test_mdl/FD1_CAN_P702_GASD_MY21_DCV_V06/GWM/PARSEDFuncGWM_ECG_FD1 ==
  PARSEDFuncGWM_ECG : Constant
  bus_creator : BusCreator  Inputs=1
  port : Outport
  wires:
  bus_creator/1 -> port/1  "PARSEDFuncGWM_ECG_FD1"
  PARSEDFuncGWM_ECG/1 -> bus_creator/1  "PARSEDFuncGWM_ECG"

== system test_mdl/FD1_CAN_P702_GASD_MY21_DCV_V06/GWM/PARSEDPhysGWM_ECGtoABS ==
  PARSEDPhysGWM_ECGtoABS : Constant
  bus_creator : BusCreator  Inputs=1
  port : Outport
  wires:
  bus_creator/1 -> port/1  "PARSEDPhysGWM_ECGtoABS"
  PARSEDPhysGWM_ECGtoABS/1 -> bus_creator/1  "PARSEDPhysGWM_ECGtoABS"

== system test_mdl/FD1_CAN_P702_GASD_MY21_DCV_V06/GWM/PARSEDPhysGWM_ECGtoCCM ==
  PARSEDPhysGWM_ECGtoCCM : Constant
  bus_creator : BusCreator  Inputs=1
  port : Outport
  wires:
  bus_creator/1 -> port/1  "PARSEDPhysGWM_ECGtoCCM"
  PARSEDPhysGWM_ECGtoCCM/1 -> bus_creator/1  "PARSEDPhysGWM_ECGtoCCM"

== system test_mdl/FD1_CAN_P702_GASD_MY21_DCV_V06/GWM/PARSEDPhysGWM_ECGtoIPMA ==
  PARSEDPhysGWM_ECGtoIPMA : Constant
  bus_creator : BusCreator  Inputs=1
  port : Outport
  wires:
  bus_creator/1 -> port/1  "PARSEDPhysGWM_ECGtoIPMA"
  PARSEDPhysGWM_ECGtoIPMA/1 -> bus_creator/1  "PARSEDPhysGWM_ECGtoIPMA"

== system test_mdl/FD1_CAN_P702_GASD_MY21_DCV_V06/GWM/PARSEDPhysGWM_ECGtoPCM ==
  PARSEDPhysGWM_ECGtoPCM : Constant
  bus_creator : BusCreator  Inputs=1
  port : Outport
  wires:
  bus_creator/1 -> port/1  "PARSEDPhysGWM_ECGtoPCM"
  PARSEDPhysGWM_ECGtoPCM/1 -> bus_creator/1  "PARSEDPhysGWM_ECGtoPCM"

== system test_mdl/FD1_CAN_P702_GASD_MY21_DCV_V06/GWM/PARSEDPhysGWM_ECGtoSODCMC ==
  PARSEDPhysGWM_ECGtoSODCMC : Constant
  bus_creator : BusCreator  Inputs=1
  port : Outport
  wires:
  bus_creator/1 -> port/1  "PARSEDPhysGWM_ECGtoSODCMC"
  PARSEDPhysGWM_ECGtoSODCMC/1 -> bus_creator/1  "PARSEDPhysGWM_ECGtoSODCMC"

== system test_mdl/FD1_CAN_P702_GASD_MY21_DCV_V06/GWM/PARSEDPhysGWM_ECGtoSODCMD ==
  PARSEDPhysGWM_ECGtoSODCMD : Constant
  bus_creator : BusCreator  Inputs=1
  port : Outport
  wires:
  bus_creator/1 -> port/1  "PARSEDPhysGWM_ECGtoSODCMD"
  PARSEDPhysGWM_ECGtoSODCMD/1 -> bus_creator/1  "PARSEDPhysGWM_ECGtoSODCMD"

== system test_mdl/FD1_CAN_P702_GASD_MY21_DCV_V06/GWM/PARSEDPhysGWM_ECGtoSODL ==
  PARSEDPhysGWM_ECGtoSODL : Constant
  bus_creator : BusCreator  Inputs=1
  port : Outport
  wires:
  bus_creator/1 -> port/1  "PARSEDPhysGWM_ECGtoSODL"
  PARSEDPhysGWM_ECGtoSODL/1 -> bus_creator/1  "PARSEDPhysGWM_ECGtoSODL"

== system test_mdl/FD1_CAN_P702_GASD_MY21_DCV_V06/GWM/PARSEDPhysGWM_ECGtoSODR ==
  PARSEDPhysGWM_ECGtoSODR : Constant
  bus_creator : BusCreator  Inputs=1
  port : Outport
  wires:
  bus_creator/1 -> port/1  "PARSEDPhysGWM_ECGtoSODR"
  PARSEDPhysGWM_ECGtoSODR/1 -> bus_creator/1  "PARSEDPhysGWM_ECGtoSODR"

== system test_mdl/FD1_CAN_P702_GASD_MY21_DCV_V06/GWM/PARSEDPhysGWMtoSOBDMC_FD1 ==
  PARSEDPhysGWM_ECGtoHPCM : Constant
  bus_creator : BusCreator  Inputs=1
  port : Outport
  wires:
  bus_creator/1 -> port/1  "PARSEDPhysGWMtoSOBDMC_FD1"
  PARSEDPhysGWM_ECGtoHPCM/1 -> bus_creator/1  "PARSEDPhysGWM_ECGtoHPCM"

== system test_mdl/FD1_CAN_P702_GASD_MY21_DCV_V06/GWM/PARSEDPushFcGWM_ECGtoABS ==
  PARSEDPhysGWM_ECG2toABS : Constant
  bus_creator : BusCreator  Inputs=1
  port : Outport
  wires:
  bus_creator/1 -> port/1  "PARSEDPushFcGWM_ECGtoABS"
  PARSEDPhysGWM_ECG2toABS/1 -> bus_creator/1  "PARSEDPhysGWM_ECG2toABS"

== system test_mdl/FD1_CAN_P702_GASD_MY21_DCV_V06/GWM/PARSEDPushFcGWM_ECGtoPCM ==
  PARSEDPhysGWM_ECG2toPCM : Constant
  bus_creator : BusCreator  Inputs=1
  port : Outport
  wires:
  bus_creator/1 -> port/1  "PARSEDPushFcGWM_ECGtoPCM"
  PARSEDPhysGWM_ECG2toPCM/1 -> bus_creator/1  "PARSEDPhysGWM_ECG2toPCM"

== system test_mdl/FD1_CAN_P702_GASD_MY21_DCV_V06/GWM/PHEV_Battery_Data1_FD1 ==
  BattAuxCnnct_B_Cmd : Constant
  bus_creator : BusCreator  Inputs=1
  port : Outport
  wires:
  bus_creator/1 -> port/1  "PHEV_Battery_Data1_FD1"
  BattAuxCnnct_B_Cmd/1 -> bus_creator/1  "BattAuxCnnct_B_Cmd"

== system test_mdl/FD1_CAN_P702_GASD_MY21_DCV_V06/GWM/ParkAid_Aud_Warn_CmdM_FD1 ==
  Cta_D_Rq : Constant
  PrkAidAcsyFront_D_RqDrv : Constant
  PrkAidAcsyRear_D_RqDrv : Constant
  PrkAidFront_D_RqDrv : Constant
  PrkAidRear_D_RqDrv : Constant
  Sod_D_Rq : Constant
  SteEffort_D_Rq : Constant
  bus_creator : BusCreator  Inputs=7
  port : Outport
  wires:
  bus_creator/1 -> port/1  "ParkAid_Aud_Warn_CmdM_FD1"
  Cta_D_Rq/1 -> bus_creator/1  "Cta_D_Rq"
  PrkAidAcsyFront_D_RqDrv/1 -> bus_creator/2  "PrkAidAcsyFront_D_RqDrv"
  PrkAidAcsyRear_D_RqDrv/1 -> bus_creator/3  "PrkAidAcsyRear_D_RqDrv"
  PrkAidFront_D_RqDrv/1 -> bus_creator/4  "PrkAidFront_D_RqDrv"
  PrkAidRear_D_RqDrv/1 -> bus_creator/5  "PrkAidRear_D_RqDrv"
  Sod_D_Rq/1 -> bus_creator/6  "Sod_D_Rq"
  SteEffort_D_Rq/1 -> bus_creator/7  "SteEffort_D_Rq"

== system test_mdl/FD1_CAN_P702_GASD_MY21_DCV_V06/GWM/Pass_Dr_Stat_FD1 ==
  BLISLEDStatPassSide : Constant
  ChildLckFdbckRp_B_Stat : Constant
  Memory_1_SwPsngr_Stat : Constant
  Memory_2_SwPsngr_Stat : Constant
  Memory_3_SwPsngr_Stat : Constant
  Pasngr_Lock_Sw_Cnt : Constant
  Pasngr_Lock_Sw_Stat : Constant
  RollCode_No_ActlPdm : Constant
  WndwPsngrSide_D_Stat : Constant
  bus_creator : BusCreator  Inputs=9
  port : Outport
  wires:
  bus_creator/1 -> port/1  "Pass_Dr_Stat_FD1"
  BLISLEDStatPassSide/1 -> bus_creator/1  "BLISLEDStatPassSide"
  ChildLckFdbckRp_B_Stat/1 -> bus_creator/2  "ChildLckFdbckRp_B_Stat"
  Memory_1_SwPsngr_Stat/1 -> bus_creator/3  "Memory_1_SwPsngr_Stat"
  Memory_2_SwPsngr_Stat/1 -> bus_creator/4  "Memory_2_SwPsngr_Stat"
  Memory_3_SwPsngr_Stat/1 -> bus_creator/5  "Memory_3_SwPsngr_Stat"
  Pasngr_Lock_Sw_Cnt/1 -> bus_creator/6  "Pasngr_Lock_Sw_Cnt"
  Pasngr_Lock_Sw_Stat/1 -> bus_creator/7  "Pasngr_Lock_Sw_Stat"
  RollCode_No_ActlPdm/1 -> bus_creator/8  "RollCode_No_ActlPdm"
  WndwPsngrSide_D_Stat/1 -> bus_creator/9  "WndwPsngrSide_D_Stat"

== system test_mdl/FD1_CAN_P702_GASD_MY21_DCV_V06/GWM/Personality_APIM_Data_FD1 ==
  CtrStkDsplyOp_D_Rq : Constant
  CtrStkFeatConfigActl : Constant
  CtrStkFeatNoActl : Constant
  CtrStkPersIndex_D_Actl : Constant
  Pers1OptIn_B_Stats : Constant
  Pers2OptIn_B_Stats : Constant
  Pers3OptIn_B_Stats : Constant
  Pers4OptIn_B_Stats : Constant
  PersStore_D_Rq : Constant
  bus_creator : BusCreator  Inputs=9
  port : Outport
  wires:
  bus_creator/1 -> port/1  "Personality_APIM_Data_FD1"
  CtrStkDsplyOp_D_Rq/1 -> bus_creator/1  "CtrStkDsplyOp_D_Rq"
  CtrStkFeatConfigActl/1 -> bus_creator/2  "CtrStkFeatConfigActl"
  CtrStkFeatNoActl/1 -> bus_creator/3  "CtrStkFeatNoActl"
  CtrStkPersIndex_D_Actl/1 -> bus_creator/4  "CtrStkPersIndex_D_Actl"
  Pers1OptIn_B_Stats/1 -> bus_creator/5  "Pers1OptIn_B_Stats"
  Pers2OptIn_B_Stats/1 -> bus_creator/6  "Pers2OptIn_B_Stats"
  Pers3OptIn_B_Stats/1 -> bus_creator/7  "Pers3OptIn_B_Stats"
  Pers4OptIn_B_Stats/1 -> bus_creator/8  "Pers4OptIn_B_Stats"
  PersStore_D_Rq/1 -> bus_creator/9  "PersStore_D_Rq"

== system test_mdl/FD1_CAN_P702_GASD_MY21_DCV_V06/GWM/Personality_BCM2_Data_FD1 ==
  AssocConfirm_D_Actl : Constant
  EmPrflKeyAssoc_D_Stat : Constant
  EmPrflNo_D_Stat : Constant
  Pers1Key_D_Stat : Constant
  Pers2Key_D_Stat : Constant
  Pers3Key_D_Stat : Constant
  Pers4Key_D_Stat : Constant
  PersConflict_D_Actl : Constant
  PersNoPos_D_Actl : Constant
  PersNo_D_Actl : Constant
  PersRecallSrc_D_Actl : Constant
  PersSetupAccessCtrl : Constant
  PersSetupRestr_D_Actl : Constant
  PersSetup_No_Actl : Constant
  RecallEvent_No_Cnt : Constant
  VehKeyActv_D_Stat : Constant
  bus_creator : BusCreator  Inputs=16
  port : Outport
  wires:
  bus_creator/1 -> port/1  "Personality_BCM2_Data_FD1"
  AssocConfirm_D_Actl/1 -> bus_creator/1  "AssocConfirm_D_Actl"
  EmPrflKeyAssoc_D_Stat/1 -> bus_creator/2  "EmPrflKeyAssoc_D_Stat"
  EmPrflNo_D_Stat/1 -> bus_creator/3  "EmPrflNo_D_Stat"
  Pers1Key_D_Stat/1 -> bus_creator/4  "Pers1Key_D_Stat"
  Pers2Key_D_Stat/1 -> bus_creator/5  "Pers2Key_D_Stat"
  Pers3Key_D_Stat/1 -> bus_creator/6  "Pers3Key_D_Stat"
  Pers4Key_D_Stat/1 -> bus_creator/7  "Pers4Key_D_Stat"
  PersConflict_D_Actl/1 -> bus_creator/8  "PersConflict_D_Actl"
  PersNoPos_D_Actl/1 -> bus_creator/9  "PersNoPos_D_Actl"
  PersNo_D_Actl/1 -> bus_creator/10  "PersNo_D_Actl"
  PersRecallSrc_D_Actl/1 -> bus_creator/11  "PersRecallSrc_D_Actl"
  PersSetupAccessCtrl/1 -> bus_creator/12  "PersSetupAccessCtrl"
  PersSetupRestr_D_Actl/1 -> bus_creator/13  "PersSetupRestr_D_Actl"
  PersSetup_No_Actl/1 -> bus_creator/14  "PersSetup_No_Actl"
  RecallEvent_No_Cnt/1 -> bus_creator/15  "RecallEvent_No_Cnt"
  VehKeyActv_D_Stat/1 -> bus_creator/16  "VehKeyActv_D_Stat"

== system test_mdl/FD1_CAN_P702_GASD_MY21_DCV_V06/GWM/Personality_Data_FD1 ==
  MsgCntrDsplyOp_D_Rq : Constant
  MsgCntrFeatConfigRq : Constant
  MsgCntrFeatNoRq : Constant
  MsgCntrPersIndex_D_Rq : Constant
  bus_creator : BusCreator  Inputs=4
  port : Outport
  wires:
  bus_creator/1 -> port/1  "Personality_Data_FD1"
  MsgCntrDsplyOp_D_Rq/1 -> bus_creator/1  "MsgCntrDsplyOp_D_Rq"
  MsgCntrFeatConfigRq/1 -> bus_creator/2  "MsgCntrFeatConfigRq"
  MsgCntrFeatNoRq/1 -> bus_creator/3  "MsgCntrFeatNoRq"
  MsgCntrPersIndex_D_Rq/1 -> bus_creator/4  "MsgCntrPersIndex_D_Rq"

== system test_mdl/FD1_CAN_P702_GASD_MY21_DCV_V06/GWM/PowerDistData_2_FD1 ==
  AirCondCluBatt_D_Falt : Constant
  AirCondCluGnd_D_Falt : Constant
  AirCondCluLife_D_Falt : Constant
  AirCondCluOpen_D_Falt : Constant
  AirCondClu_D_Stat : Constant
  BattChlrLifeLim_D_Falt : Constant
  BattChlrOpnCirct_D_Falt : Constant
  BattChlrShrtBatt_D_Falt : Constant
  BattChlrShrtGrnd_D_Falt : Constant
  BattTracLifeLim_D_Falt : Constant
  BattTracLow_D_Falt : Constant
  BattTracOpnCirct_D_Falt : Constant
  BattTracShrtBatt_D_Falt : Constant
  BattTracShrtGrnd_D_Falt : Constant
  bus_creator : BusCreator  Inputs=14
  port : Outport
  wires:
  bus_creator/1 -> port/1  "PowerDistData_2_FD1"
  AirCondCluBatt_D_Falt/1 -> bus_creator/1  "AirCondCluBatt_D_Falt"
  AirCondCluGnd_D_Falt/1 -> bus_creator/2  "AirCondCluGnd_D_Falt"
  AirCondCluLife_D_Falt/1 -> bus_creator/3  "AirCondCluLife_D_Falt"
  AirCondCluOpen_D_Falt/1 -> bus_creator/4  "AirCondCluOpen_D_Falt"
  AirCondClu_D_Stat/1 -> bus_creator/5  "AirCondClu_D_Stat"
  BattChlrLifeLim_D_Falt/1 -> bus_creator/6  "BattChlrLifeLim_D_Falt"
  BattChlrOpnCirct_D_Falt/1 -> bus_creator/7  "BattChlrOpnCirct_D_Falt"
  BattChlrShrtBatt_D_Falt/1 -> bus_creator/8  "BattChlrShrtBatt_D_Falt"
  BattChlrShrtGrnd_D_Falt/1 -> bus_creator/9  "BattChlrShrtGrnd_D_Falt"
  BattTracLifeLim_D_Falt/1 -> bus_creator/10  "BattTracLifeLim_D_Falt"
  BattTracLow_D_Falt/1 -> bus_creator/11  "BattTracLow_D_Falt"
  BattTracOpnCirct_D_Falt/1 -> bus_creator/12  "BattTracOpnCirct_D_Falt"
  BattTracShrtBatt_D_Falt/1 -> bus_creator/13  "BattTracShrtBatt_D_Falt"
  BattTracShrtGrnd_D_Falt/1 -> bus_creator/14  "BattTracShrtGrnd_D_Falt"

== system test_mdl/FD1_CAN_P702_GASD_MY21_DCV_V06/GWM/PowerDist_Data1_FD1 ==
  BattChlrSov_D_Stat : Constant
  BattTracClntVlv_D_Stat : Constant
  CabnEvapSovFront_D_Stat : Constant
  bus_creator : BusCreator  Inputs=3
  port : Outport
  wires:
  bus_creator/1 -> port/1  "PowerDist_Data1_FD1"
  BattChlrSov_D_Stat/1 -> bus_creator/1  "BattChlrSov_D_Stat"
  BattTracClntVlv_D_Stat/1 -> bus_creator/2  "BattTracClntVlv_D_Stat"
  CabnEvapSovFront_D_Stat/1 -> bus_creator/3  "CabnEvapSovFront_D_Stat"

== system test_mdl/FD1_CAN_P702_GASD_MY21_DCV_V06/GWM/Power_Liftgate_Stat_FD1 ==
  DrLckCnt_No_ActlTgate : Constant
  DrTGate_D_Rq : Constant
  DrTgateChime2_D_Rq : Constant
  Power_Liftgate_Mode_Stt : Constant
  PwLftgtIntSw_B_Stat : Constant
  bus_creator : BusCreator  Inputs=5
  port : Outport
  wires:
  bus_creator/1 -> port/1  "Power_Liftgate_Stat_FD1"
  DrLckCnt_No_ActlTgate/1 -> bus_creator/1  "DrLckCnt_No_ActlTgate"
  DrTGate_D_Rq/1 -> bus_creator/2  "DrTGate_D_Rq"
  DrTgateChime2_D_Rq/1 -> bus_creator/3  "DrTgateChime2_D_Rq"
  Power_Liftgate_Mode_Stt/1 -> bus_creator/4  "Power_Liftgate_Mode_Stt"
  PwLftgtIntSw_B_Stat/1 -> bus_creator/5  "PwLftgtIntSw_B_Stat"

== system test_mdl/FD1_CAN_P702_GASD_MY21_DCV_V06/GWM/RCMSerialNumber_FD1 ==
  RCMSerialNoByte{1..8} (8 alike) : Constant
  bus_creator : BusCreator  Inputs=8
  port : Outport
  wires:
  bus_creator/1 -> port/1  "RCMSerialNumber_FD1"
  RCMSerialNoByte1/1 -> bus_creator/1  "RCMSerialNoByte1"
  RCMSerialNoByte2/1 -> bus_creator/2  "RCMSerialNoByte2"
  RCMSerialNoByte3/1 -> bus_creator/3  "RCMSerialNoByte3"
  RCMSerialNoByte4/1 -> bus_creator/4  "RCMSerialNoByte4"
  RCMSerialNoByte5/1 -> bus_creator/5  "RCMSerialNoByte5"
  RCMSerialNoByte6/1 -> bus_creator/6  "RCMSerialNoByte6"
  RCMSerialNoByte7/1 -> bus_creator/7  "RCMSerialNoByte7"
  RCMSerialNoByte8/1 -> bus_creator/8  "RCMSerialNoByte8"

== system test_mdl/FD1_CAN_P702_GASD_MY21_DCV_V06/GWM/RCMStatusMessage2_FD1 ==
  EDRTriggerEvntSync : Constant
  FirstRowBuckleDriver : Constant
  FirstRowBuckleMid : Constant
  FirstRowBucklePsngr : Constant
  PassRstrnInd_Req : Constant
  PsngrFrntDetct_D_Actl : Constant
  RILReq : Constant
  RstrnImpactEvntStatus : Constant
  SecondRowBuckleDriver : Constant
  SecondRowBuckleMid : Constant
  SecondRowBucklePsngr : Constant
  bus_creator : BusCreator  Inputs=11
  port : Outport
  wires:
  bus_creator/1 -> port/1  "RCMStatusMessage2_FD1"
  EDRTriggerEvntSync/1 -> bus_creator/1  "EDRTriggerEvntSync"
  FirstRowBuckleDriver/1 -> bus_creator/2  "FirstRowBuckleDriver"
  FirstRowBuckleMid/1 -> bus_creator/3  "FirstRowBuckleMid"
  FirstRowBucklePsngr/1 -> bus_creator/4  "FirstRowBucklePsngr"
  PassRstrnInd_Req/1 -> bus_creator/5  "PassRstrnInd_Req"
  PsngrFrntDetct_D_Actl/1 -> bus_creator/6  "PsngrFrntDetct_D_Actl"
  RILReq/1 -> bus_creator/7  "RILReq"
  RstrnImpactEvntStatus/1 -> bus_creator/8  "RstrnImpactEvntStatus"
  SecondRowBuckleDriver/1 -> bus_creator/9  "SecondRowBuckleDriver"
  SecondRowBuckleMid/1 -> bus_creator/10  "SecondRowBuckleMid"
  SecondRowBucklePsngr/1 -> bus_creator/11  "SecondRowBucklePsngr"

== system test_mdl/FD1_CAN_P702_GASD_MY21_DCV_V06/GWM/SmartChargingData_ECG_1 ==
  ScLocDelete_B_RqCld : Constant
  ScLocId_No_RqCld : Constant
  ScLocLattDeg_An_RqCld : Constant
  ScLocLattFrct_An_RqCld : Constant
  ScLocLattPostv_B_RqCld : Constant
  ScLocLongDeg_An_RqCld : Constant
  ScLocLongFrct_An_RqCld : Constant
  ScLocLongPostv_B_RqCld : Constant
  bus_creator : BusCreator  Inputs=8
  port : Outport
  wires:
  bus_creator/1 -> port/1  "SmartChargingData_ECG_1"
  ScLocDelete_B_RqCld/1 -> bus_creator/1  "ScLocDelete_B_RqCld"
  ScLocId_No_RqCld/1 -> bus_creator/2  "ScLocId_No_RqCld"
  ScLocLattDeg_An_RqCld/1 -> bus_creator/3  "ScLocLattDeg_An_RqCld"
  ScLocLattFrct_An_RqCld/1 -> bus_creator/4  "ScLocLattFrct_An_RqCld"
  ScLocLattPostv_B_RqCld/1 -> bus_creator/5  "ScLocLattPostv_B_RqCld"
  ScLocLongDeg_An_RqCld/1 -> bus_creator/6  "ScLocLongDeg_An_RqCld"
  ScLocLongFrct_An_RqCld/1 -> bus_creator/7  "ScLocLongFrct_An_RqCld"
  ScLocLongPostv_B_RqCld/1 -> bus_creator/8  "ScLocLongPostv_B_RqCld"

== system test_mdl/FD1_CAN_P702_GASD_MY21_DCV_V06/GWM/SmartChargingData_ECG_2 ==
  ScChrgDurSet_D_RqCld : Constant
  ScChrgDur_T_RqCld : Constant
  ScChrgPrfl_No_RqCld : Constant
  ScChrgToPc_Pc_RqCld : Constant
  ScDayOfWeekId_D_RqCld : Constant
  ScLocRdius_L_RqCld : Constant
  ScLocSetId_No_RqCld : Constant
  bus_creator : BusCreator  Inputs=7
  port : Outport
  wires:
  bus_creator/1 -> port/1  "SmartChargingData_ECG_2"
  ScChrgDurSet_D_RqCld/1 -> bus_creator/1  "ScChrgDurSet_D_RqCld"
  ScChrgDur_T_RqCld/1 -> bus_creator/2  "ScChrgDur_T_RqCld"
  ScChrgPrfl_No_RqCld/1 -> bus_creator/3  "ScChrgPrfl_No_RqCld"
  ScChrgToPc_Pc_RqCld/1 -> bus_creator/4  "ScChrgToPc_Pc_RqCld"
  ScDayOfWeekId_D_RqCld/1 -> bus_creator/5  "ScDayOfWeekId_D_RqCld"
  ScLocRdius_L_RqCld/1 -> bus_creator/6  "ScLocRdius_L_RqCld"
  ScLocSetId_No_RqCld/1 -> bus_creator/7  "ScLocSetId_No_RqCld"

== system test_mdl/FD1_CAN_P702_GASD_MY21_DCV_V06/GWM/SmartChargingData_ECG_3 ==
  AirAmb_Te_ActlCld : Constant
  ChrgToPcEdit_Pc_RqCld : Constant
  GoTEditHr_T_RqCld : Constant
  GoTEditMnte_T_RqCld : Constant
  PrcondEdit_D_RqCld : Constant
  ScChrgrPwMax_Pw_RqCld : Constant
  ScEnbl_D_RqCld : Constant
  ScFreshDataEnbl_B_Rq : Constant
  ScLocPwId_No_RqCld : Constant
  ScMnSoc_Pc_RqCld : Constant
  bus_creator : BusCreator  Inputs=10
  port : Outport
  wires:
  bus_creator/1 -> port/1  "SmartChargingData_ECG_3"
  AirAmb_Te_ActlCld/1 -> bus_creator/1  "AirAmb_Te_ActlCld"
  ChrgToPcEdit_Pc_RqCld/1 -> bus_creator/2  "ChrgToPcEdit_Pc_RqCld"
  GoTEditHr_T_RqCld/1 -> bus_creator/3  "GoTEditHr_T_RqCld"
  GoTEditMnte_T_RqCld/1 -> bus_creator/4  "GoTEditMnte_T_RqCld"
  PrcondEdit_D_RqCld/1 -> bus_creator/5  "PrcondEdit_D_RqCld"
  ScChrgrPwMax_Pw_RqCld/1 -> bus_creator/6  "ScChrgrPwMax_Pw_RqCld"
  ScEnbl_D_RqCld/1 -> bus_creator/7  "ScEnbl_D_RqCld"
  ScFreshDataEnbl_B_Rq/1 -> bus_creator/8  "ScFreshDataEnbl_B_Rq"
  ScLocPwId_No_RqCld/1 -> bus_creator/9  "ScLocPwId_No_RqCld"
  ScMnSoc_Pc_RqCld/1 -> bus_creator/10  "ScMnSoc_Pc_RqCld"
